simulink model "Plant_IM"  (R2021a)
settings: Solver=FixedStepAuto  StartTime=0.0  StopTime=10.0  RelTol=1e-3
settings Model: Creator=Mehra  LastModifiedBy=Mehra
settings DataIOCC: SaveOutput=off  SaveTime=off

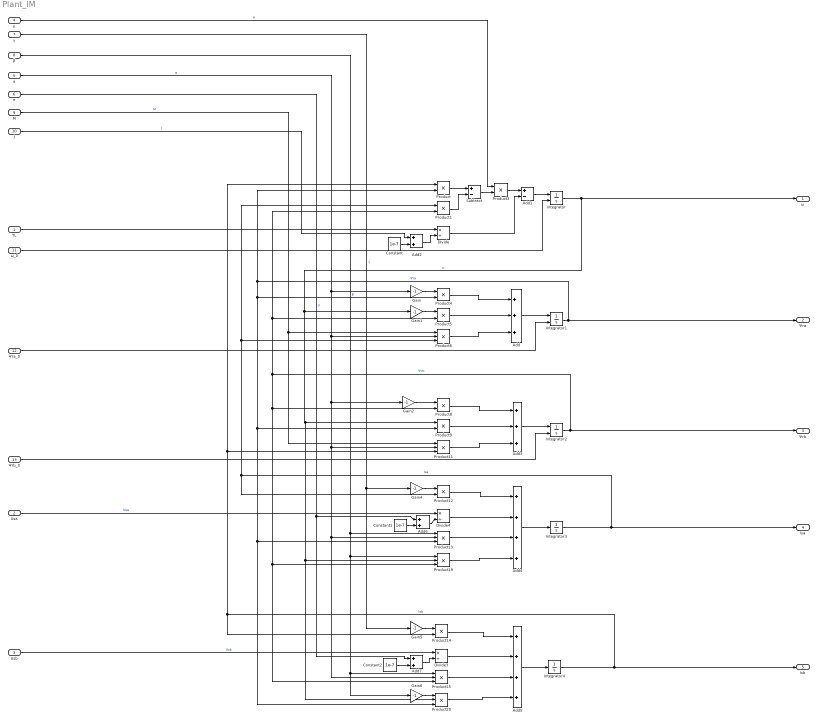
== system Plant_IM ==
  TL : Inport  OutDataTypeStr=double  PortDimensions=1
  Usa : Inport  Port=2  OutDataTypeStr=double  PortDimensions=1  SampleTime=0
  Usb : Inport  Port=3  OutDataTypeStr=double  PortDimensions=1  SampleTime=0
  µ : Inport  Port=4  OutDataTypeStr=double  PortDimensions=1
  α : Inport  Port=5  OutDataTypeStr=double  PortDimensions=1
  σ : Inport  Port=6  OutDataTypeStr=double  PortDimensions=1
  γ : Inport  Port=7  OutDataTypeStr=double  PortDimensions=1
  β : Inport  Port=8  OutDataTypeStr=double  PortDimensions=1
  M : Inport  Port=9  OutDataTypeStr=double  PortDimensions=1
  J : Inport  Port=10  OutDataTypeStr=double  PortDimensions=1
  ω_0 : Inport  Port=11
  Ψra_0 : Inport  Port=12
  Ψrb_0 : Inport  Port=13
  Add : Sum  Inputs=+++
  Add1 : Sum  Inputs=+-
  Add2 : Sum
  Add3 : Sum  Inputs=+++
  Add4 : Sum  Inputs=++++
  Add5 : Sum  Inputs=++++
  Add6 : Sum
  Add7 : Sum
  Constant : Constant  Value=1e-7
  Constant1 : Constant  Value=1e-7
  Constant2 : Constant  Value=1e-7
  Divide : Product  Inputs=*/
  Divide3 : Product  Inputs=*/
  Divide4 : Product  Inputs=*/
  Gain{,1..2,4..6} (6 alike) : Gain  Gain=-1
  Integrator : Integrator  InitialConditionSource=external
  Integrator1 : Integrator  InitialConditionSource=external  UpperSaturationLimit=1000
  Integrator2 : Integrator  InitialConditionSource=external  UpperSaturationLimit=1000
  Integrator3 : Integrator
  Integrator4 : Integrator
  Product{,1,3..5,8..9,12,14} (9 alike) : Product
  Product{6,11,13,15,19..20} (6 alike) : Product  Inputs=3
  Subtract : Sum  Inputs=+-
  ω : Outport  OutDataTypeStr=double  PortDimensions=1  SampleTime=0
  Ψra : Outport  Port=2  OutDataTypeStr=double  PortDimensions=1  SampleTime=0
  Ψrb : Outport  Port=3  OutDataTypeStr=double  PortDimensions=1  SampleTime=0
  Isa : Outport  Port=4  OutDataTypeStr=double  PortDimensions=1  SampleTime=0
  Isb : Outport  Port=5  OutDataTypeStr=double  PortDimensions=1  SampleTime=0
  wires:
  Add/1 -> Integrator1/1
  Integrator1/1 -> Product/2, Product9/2, Product13/3, Product20/3, Product4/2, Ψra/1  "Ψra"
  Integrator/1 -> ω/1, Gain1/1, Product20/2, Product19/2, Product9/1  "ω"
  Product6/1 -> Add/3
  Product8/1 -> Add3/1
  Integrator4/1 -> Product14/2, Product/1, Product11/3, Isb/1  "Isb"
  Gain5/1 -> Product14/1
  Integrator3/1 -> Product12/2, Product1/1, Product6/3, Isa/1  "Isa"
  Product11/1 -> Add3/3
  Product3/1 -> Add1/1
  Integrator2/1 -> Product5/2, Product1/2, Product8/2, Product15/3, Product19/3, Ψrb/1  "Ψrb"
  Product15/1 -> Add5/3
  Product4/1 -> Add/1
  α/1 -> Gain/1, Gain2/1, Product11/2, Product15/2, Product13/2, Product6/2  "α"
  Gain1/1 -> Product5/1
  Product14/1 -> Add5/1
  Add4/1 -> Integrator3/1
  µ/1 -> Product3/1  "µ"
  Add5/1 -> Integrator4/1
  Add3/1 -> Integrator2/1
  Gain/1 -> Product4/1
  Product9/1 -> Add3/2
  σ/1 -> Add7/1, Add6/1  "σ"
  Gain2/1 -> Product8/1
  Usa/1 -> Divide4/1  "Usa"
  Gain4/1 -> Product12/1
  Product5/1 -> Add/2
  TL/1 -> Divide/1
  Gain6/1 -> Product20/1
  γ/1 -> Gain5/1, Gain4/1  "γ"
  Subtract/1 -> Product3/2
  Divide4/1 -> Add4/2
  Divide/1 -> Add1/2
  Usb/1 -> Divide3/1  "Usb"
  Product1/1 -> Subtract/2
  Product/1 -> Subtract/1
  Product20/1 -> Add5/4
  Divide3/1 -> Add5/2
  Product12/1 -> Add4/1
  Add1/1 -> Integrator/1
  β/1 -> Gain6/1, Product15/1, Product19/1, Product13/1  "β"
  Product19/1 -> Add4/4
  M/1 -> Product11/1, Product6/1  "M"
  Product13/1 -> Add4/3
  ω_0/1 -> Integrator/2
  Ψra_0/1 -> Integrator1/2
  Ψrb_0/1 -> Integrator2/2
  Add2/1 -> Divide/2
  J/1 -> Add2/1  "J"
  Constant/1 -> Add2/2
  Constant1/1 -> Add6/2
  Add6/1 -> Divide4/2
  Add7/1 -> Divide3/2
  Constant2/1 -> Add7/2
